simulink model "Lazurit_zarud_"  (R2018b)
settings: Solver=VariableStepAuto  StartTime=0.0  StopTime=1  RelTol=1e-3
undefined symbols (not defined in the file): Cout_c, Cout_filter_c, Cout_filter_r, Cout_r, Czpt_c, Czpt_r, DiscIntNeverNeededParam, f, L_l, L_r, Lzpt_l, Lzpt_r, Rout, Ul, Uout
libraries: powerlib x36, dspstat3 x15, powerlib_meascontrol x8, simulink x4, simulink_extras x4, peRmsMeasurement x4
settings Model: Creator=VID Company  LastModifiedBy=VID Company

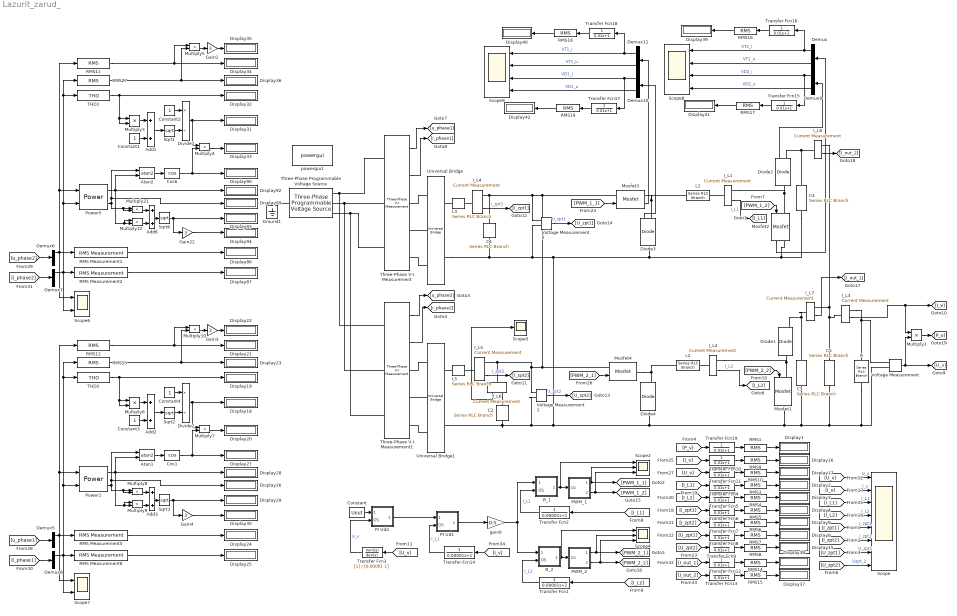
== system Lazurit_zarud_ ==
  Add{1..3,6} (4 alike) : Sum
  Atan1 : Trigonometry  Operator=atan2
  Atan2 : Trigonometry  Operator=atan2
  C1 : powerlib/Elements/Series RLC Branch  LConnTagsString=__new0  RConnTagsString=__new0  BranchType=RC  Resistance=Czpt_r  Inductance=1e-3  SetiL0=off  InitialCurrent=0  Capacitance=Czpt_c  Setx0=on  InitialVoltage=Uzpt  Measurements=Branch voltage
      settings: SourceProductName=Simscape Electrical
  C2 : powerlib/Elements/Series RLC Branch  LConnTagsString=__new0  RConnTagsString=__new0  BranchType=RC  Resistance=Czpt_r  Inductance=1e-3  SetiL0=off  InitialCurrent=0  Capacitance=Czpt_c  Setx0=on  InitialVoltage=Uzpt  Measurements=Branch voltage
      settings: SourceProductName=Simscape Electrical
  C3 : powerlib/Elements/Series RLC Branch  LConnTagsString=__new0  RConnTagsString=__new0  BranchType=RC  Resistance=Cout_r  Inductance=1e-3  SetiL0=off  InitialCurrent=0  Capacitance=Cout_c  Setx0=on  InitialVoltage=0  Measurements=Branch voltage
      settings: SourceProductName=Simscape Electrical
  C4 : powerlib/Elements/Series RLC Branch  LConnTagsString=__new0  RConnTagsString=__new0  BranchType=RC  Resistance=Cout_r  Inductance=1e-3  SetiL0=off  InitialCurrent=0  Capacitance=Cout_c  Setx0=on  InitialVoltage=0  Measurements=Branch voltage
      settings: SourceProductName=Simscape Electrical
  C5 : powerlib/Elements/Series RLC Branch  LConnTagsString=__new0  RConnTagsString=__new0  BranchType=RC  Resistance=Cout_filter_r  Inductance=1e-3  SetiL0=off  InitialCurrent=0  Capacitance=Cout_filter_c  Setx0=on  InitialVoltage=0  Measurements=Branch voltage
      settings: SourceProductName=Simscape Electrical
  Constant : Constant  Value=Uout
  Constant{1..4} (4 alike) : Constant
  Cos1 : Trigonometry  Operator=cos
  Cos6 : Trigonometry  Operator=cos
  Demux{,9..11} (4 alike) : Demux  Outputs=2
  Demux{5..8} (4 alike) : Demux  Outputs=3
  Diode{1..4} (4 alike) : powerlib/Power Electronics/Diode  Ron=0.001  Lon=0  Vf=0.8  IC=0  UseSnubber=off  Rs=500  Cs=250e-9  Measurements=on
      settings: SourceProductName=Simscape Electrical
  Display{1..4,8..9,15..42,86..87,89..90,92..94} (41 alike) : Display
  Divide1 : Product  Inputs=*/
  Divide2 : Product  Inputs=*/
  Gain{1,3..4,22} (4 alike) : Gain  Gain=3
  Ground1 : powerlib/Elements/Ground  LConnTagsString=a
  I_L{1..8} (8 alike) : powerlib/Measurements/Current Measurement  PhasorSimulation=off  OutputType=Complex  PSBequivalent=0
      settings: SourceProductName=Simscape Electrical
  L1 : powerlib/Elements/Series RLC Branch  LConnTagsString=__new0  RConnTagsString=__new0  BranchType=RL  Resistance=L_r  Inductance=L_l  SetiL0=off  InitialCurrent=0  Capacitance=1e-6  Setx0=off  InitialVoltage=0  Measurements=None
      settings: SourceProductName=Simscape Electrical
  L2 : powerlib/Elements/Series RLC Branch  LConnTagsString=__new0  RConnTagsString=__new0  BranchType=RL  Resistance=L_r  Inductance=L_l  SetiL0=off  InitialCurrent=0  Capacitance=1e-6  Setx0=off  InitialVoltage=0  Measurements=None
      settings: SourceProductName=Simscape Electrical
  L3 : powerlib/Elements/Series RLC Branch  LConnTagsString=__new0  RConnTagsString=__new0  BranchType=RL  Resistance=Lzpt_r  Inductance=Lzpt_l  SetiL0=off  InitialCurrent=0  Capacitance=1e-6  Setx0=off  InitialVoltage=0  Measurements=None
      settings: SourceProductName=Simscape Electrical
  L5 : powerlib/Elements/Series RLC Branch  LConnTagsString=__new0  RConnTagsString=__new0  BranchType=RL  Resistance=Lzpt_r  Inductance=Lzpt_l  SetiL0=off  InitialCurrent=0  Capacitance=1e-6  Setx0=off  InitialVoltage=0  Measurements=None
      settings: SourceProductName=Simscape Electrical
  Mosfet1 : powerlib/Power Electronics/Mosfet  Ron=1e-6  Lon=0  Rd=1e-6  Vfd=0  IC=0  Rs=1e5  Cs=inf  Measurements=off
      settings: SourceProductName=Simscape Electrical
  Mosfet2 : powerlib/Power Electronics/Mosfet  Ron=1e-6  Lon=0  Rd=1e-6  Vfd=0  IC=0  Rs=1e5  Cs=inf  Measurements=on
      settings: SourceProductName=Simscape Electrical
  Mosfet3 : powerlib/Power Electronics/Mosfet  Ron=1e-6  Lon=0  Rd=1e-6  Vfd=0  IC=0  Rs=1e5  Cs=inf  Measurements=on
      settings: SourceProductName=Simscape Electrical
  Mosfet4 : powerlib/Power Electronics/Mosfet  Ron=1e-6  Lon=0  Rd=1e-6  Vfd=0  IC=0  Rs=1e5  Cs=inf  Measurements=off
      settings: SourceProductName=Simscape Electrical
  Multiply{1,3..10,21..22} (11 alike) : Product
  PI Ud1 : Subsystem
  PI Ud2 : Subsystem
  PWM_1 : Subsystem
  PWM_2 : Subsystem
  Power1 : powerlib_meascontrol/Measurements/Power  Freq=50  Vinit=[1, 0]  Iinit=[1, 0]  Ts=0
      settings: SourceProductName=Simscape Power Systems
  Power5 : powerlib_meascontrol/Measurements/Power  Freq=50  Vinit=[1, 0]  Iinit=[1, 0]  Ts=0
      settings: SourceProductName=Simscape Power Systems
  R : powerlib/Elements/Series RLC Branch  LConnTagsString=__new0  RConnTagsString=__new0  BranchType=R  Resistance=Rout  Inductance=1e-3  SetiL0=off  InitialCurrent=0  Capacitance=6000e-6  Setx0=off  InitialVoltage=0  Measurements=None
  RMS Measurement{1..2,5,8} (4 alike) : peRmsMeasurement/RMS Measurement  LabelModeActiveChoice=Harmonic  F=50  SpecifyHarmonics=on  K=[1]  Ts=0
  RMS{1,3..10,14..19} (15 alike) : dspstat3/RMS  run=off  directionMode=Each column  dimension=1  InputProcessing=Columns as channels (frame based)  reset_popup=None
  RMS{11..13,27} (4 alike) : powerlib_meascontrol/Measurements/RMS  TrueRMS=on  Freq=50  RMSInit=0  Ts=0
  R_1 : Subsystem
  R_2 : Subsystem
  Scope : Scope  NumInputPorts=8
  Scope2 : Scope  NumInputPorts=3
  Scope4 : Scope  NumInputPorts=3
  Scope5 : Scope
  Scope6 : Scope  NumInputPorts=2
  Scope7 : Scope  NumInputPorts=2
  Scope8 : Scope  NumInputPorts=4
  Scope9 : Scope  NumInputPorts=4
  Sqrt{1..3,6} (4 alike) : Sqrt  SaturateOnIntegerOverflow=on
  THD1 : powerlib_meascontrol/Measurements/THD  Freq=50  Ts=0
  THD2 : powerlib_meascontrol/Measurements/THD  Freq=50  Ts=0
  Three-Phase Programmable Voltage Source : powerlib/Electrical Sources/Three-Phase Programmable Voltage Source  PositiveSequence=[Ul 0 50]  VariationEntity=None  VariationType=Table of time-amplitude pairs  VariationTypeAlt=Step  VariationStep=0.5  VariationRate=10  VariationMagnitude=0.3  VariationFrequency=2  VariationTiming=[1 2]  VariationPhaseA=off  Amplitudes=[1 0.8 1.2 1.0]  TimeValues=[0 0.1 0.15 0.2]  HarmonicGeneration=off  HarmonicA=[3 0.2 -25 0]  HarmonicB=[2 0.15 35 2]  Timing="[0.05  3]"  BusType=swing  Pref=0  Qref=0  Qmin=-inf  Qmax=inf
  Three-Phase V-I Measurement : powerlib/Measurements/Three-Phase V-I Measurement  VoltageMeasurement=phase-to-ground  SetLabelV=off  LabelV=Vabc  Vpu=off  VpuLL=off  CurrentMeasurement=yes  SetLabelI=off  LabelI=Iabc  Ipu=off  Pbase=100e6  Vbase=500e3  OutputType=Complex  PhasorSimulation=off  PSBequivalent=0
  Three-Phase V-I Measurement1 : powerlib/Measurements/Three-Phase V-I Measurement  VoltageMeasurement=phase-to-ground  SetLabelV=off  LabelV=Vabc  Vpu=off  VpuLL=off  CurrentMeasurement=yes  SetLabelI=off  LabelI=Iabc  Ipu=off  Pbase=100e6  Vbase=500e3  OutputType=Complex  PhasorSimulation=off  PSBequivalent=0
  Transfer Fcn{1..3,14} (4 alike) : TransferFcn  Denominator=[0.00001 1]
  Transfer Fcn{4..13,15..19} (15 alike) : TransferFcn  Denominator=[0.01 1]
  Universal Bridge : powerlib/Power Electronics/Universal Bridge  Arms=3  SnubberResistance=1e5  SnubberCapacitance=inf  Device=Diodes  Ron=Vd_r  Lon=0  ForwardVoltages="[  0  0  ]"  ForwardVoltage=Vd_v  GTOparameters=[ 10e-6 , 20e-6 ]  IGBTparameters=[ 1e-6 , 2e-6 ]  Measurements=None  Measurements_2=None  converterType=Rectifier
  Universal Bridge1 : powerlib/Power Electronics/Universal Bridge  Arms=3  SnubberResistance=1e5  SnubberCapacitance=inf  Device=Diodes  Ron=Vd_r  Lon=0  ForwardVoltages="[  0  0  ]"  ForwardVoltage=Vd_v  GTOparameters=[ 10e-6 , 20e-6 ]  IGBTparameters=[ 1e-6 , 2e-6 ]  Measurements=None  Measurements_2=None  converterType=Rectifier
  Voltage Measurement : powerlib/Measurements/Voltage Measurement  PhasorSimulation=off  OutputType=Complex  PSBequivalent=0
  Voltage Measurement1 : powerlib/Measurements/Voltage Measurement  PhasorSimulation=off  OutputType=Complex  PSBequivalent=0
  Voltage Measurement2 : powerlib/Measurements/Voltage Measurement  PhasorSimulation=off  OutputType=Complex  PSBequivalent=0
  gain6 : Gain  Gain=0.5  SaturateOnIntegerOverflow=on  OutDataTypeStr=Inherit: Same as input  ParamDataTypeStr=Inherit: Same as input
  powergui1 : powerlib/powergui  Priority=1  SimulationMode=Discrete  SampleTime=1e-6  frequency=60  Iterations=50  frequencyindice=50  Pbase=100e6  ErrMax=1e-4  UnitsV=kV  UnitsW=MW  buscounter=0  FunctionMessages=off  echomessages=off  EnableUseOfTLC=off  CurrentSourceSwitches=off  DisableSnubberDevices=off  DisableRonSwitches=off  DisableVfSwitches=off  DisplayEquations=off  SolverType=Tustin/Backward Euler (TBE)  Interpol=off  ExternalGateDelay=off  methode=off  Ts=100  x0status=blocks  SPID=on  SwTol=0  HookPort=off  RestoreLinks=warning  ResistiveCurrentMeasurement=off  Frange=[0:2:500]  Ylog=off  Xlog=on  ShowGrid=off  save=off  variable=ZData  structure=logsout  ZoomFFT=off  StartTime=0.1  cycles=30  DisplayStyle=2  fundamental=50  FreqAxis=off  MaxFrequency=1000  frequencyindicesteady=1  RmsSteady=1  display=off
  wires:
  Three-Phase V-I Measurement/1 -> [u_phase1]
  Three-Phase V-I Measurement1/1 -> [u_phase2]
  Three-Phase V-I Measurement/2 -> [i_phase1]
  Three-Phase V-I Measurement1/2 -> [i_phase2]
  R_1/1(Out) -> Scope2/1, PWM_1/1(Uz)
  Transfer Fcn2/1 -> R_1/2(OS)  "I_L1"
  Transfer Fcn1/1 -> R_2/2(OS)  "I_L2"
  gain6/1 -> R_1/1(Zad), R_2/1(Zad)
  R_2/1(Out) -> Scope4/1, PWM_2/1(Uz)
  Constant/1 -> PI Ud2/1(Zad)
  Transfer Fcn3/1 -> PI Ud2/2(OS)  "U_v"
  I_L1/1 -> [I_L1]  "I_L1"
  PWM_1/1(CH1) -> Scope2/2, [PWM_1_1]
  [PWM_1_2] -> Mosfet2/1
  [I_L1] -> Transfer Fcn2/1
  PWM_2/1(CH1) -> Scope4/2, [PWM_2_1]
  I_L2/1 -> [I_L2]  "I_L2"
  [I_L2] -> Transfer Fcn1/1
  [PWM_2_2] -> Mosfet1/1
  Voltage Measurement/1 -> [U_v], Multiply1/2
  [U_v] -> Transfer Fcn3/1
  [U_v] -> Scope/1  "U_v"
  [I_L1] -> Scope/3  "I_L1"
  [I_L2] -> Scope/4  "I_L2"
  I_L3/1 -> [I_v], Multiply1/1
  [I_v] -> Scope/2  "I_v"
  I_L5/1 -> [I_zpt2]  "I_zpt2"
  I_L4/1 -> [I_zpt1]  "I_zpt1"
  [I_zpt1] -> Scope/5  "I_zpt1"
  [I_zpt2] -> Scope/6  "I_zpt2"
  Voltage Measurement1/1 -> [U_zpt2]  "U_zpt2"
  Voltage Measurement2/1 -> [U_zpt1]  "U_zpt1"
  [U_zpt1] -> Scope/7  "U_zpt1"
  [U_zpt2] -> Scope/8  "Uzpt_2"
  Multiply1/1 -> [P_v]
  [I_L1] -> Transfer Fcn4/1
  [I_L2] -> Transfer Fcn5/1
  [I_zpt1] -> Transfer Fcn6/1
  [I_zpt2] -> Transfer Fcn7/1
  [U_zpt1] -> Transfer Fcn8/1
  [U_zpt2] -> Transfer Fcn9/1
  RMS3/1 -> Display2/1
  RMS4/1 -> Display3/1
  RMS5/1 -> Display4/1
  RMS6/1 -> Display9/1
  RMS7/1 -> Display8/1
  RMS8/1 -> Display15/1
  Transfer Fcn4/1 -> RMS3/1
  Transfer Fcn5/1 -> RMS4/1
  Transfer Fcn6/1 -> RMS5/1
  Transfer Fcn7/1 -> RMS6/1
  Transfer Fcn8/1 -> RMS7/1
  Transfer Fcn9/1 -> RMS8/1
  PWM_1/2(CH2) -> Scope2/3, [PWM_1_2]
  [PWM_1_1] -> Mosfet3/1
  PWM_2/2(CH2) -> [PWM_2_2], Scope4/3
  [PWM_2_1] -> Mosfet4/1
  Transfer Fcn10/1 -> RMS9/1
  RMS9/1 -> Display16/1
  [I_v] -> Transfer Fcn10/1
  Transfer Fcn11/1 -> RMS10/1
  RMS10/1 -> Display17/1
  [U_v] -> Transfer Fcn11/1
  I_L6/1 -> Scope5/1
  Multiply3/1 -> Add1/1
  Multiply5/1 -> Gain1/1
  Add1/1 -> Sqrt1/1
  Multiply4/1 -> Display33/1
  Constant1/1 -> Add1/2
  Constant2/1 -> Divide1/1
  Power5/1 -> Atan2/2, Multiply22/1, Multiply22/2, Display92/1
  Cos6/1 -> Multiply4/2, Display90/1
  RMS Measurement1/1 -> Display86/1
  Demux7/1 -> Scope6/2, RMS Measurement2/1, THD1/1, RMS27/1, Power5/2
  [i_phase2] -> Demux7/1
  Power5/2 -> Atan2/1, Display89/1, Multiply21/2, Multiply21/1
  [i_phase1] -> Demux8/1
  RMS11/1 -> Multiply5/1, Display34/1
  Sqrt2/1 -> Divide2/2
  Gain1/1 -> Display35/1
  Multiply21/1 -> Add6/1
  Divide1/1 -> Multiply4/1, Display31/1
  Demux6/1 -> Scope6/1, RMS Measurement1/1, RMS11/1, Power5/1
  Cos1/1 -> Multiply7/2, Display27/1
  Gain3/1 -> Display22/1
  Multiply8/1 -> Add3/1
  Multiply9/1 -> Add3/2
  Sqrt6/1 -> Display93/1, Gain22/1
  Sqrt1/1 -> Divide1/2
  Divide2/1 -> Multiply7/1, Display18/1
  [u_phase2] -> Demux6/1
  Atan2/1 -> Cos6/1
  Add6/1 -> Sqrt6/1
  RMS Measurement8/1 -> Display25/1
  Atan1/1 -> Cos1/1
  RMS Measurement5/1 -> Display24/1
  Demux8/1 -> Scope7/2, RMS Measurement8/1, THD2/1, RMS13/1, Power1/2
  [u_phase1] -> Demux5/1
  Constant4/1 -> Divide2/1
  RMS13/1 -> Multiply10/2, Display23/1
  RMS Measurement2/1 -> Display87/1
  RMS12/1 -> Multiply10/1, Display21/1
  Multiply6/1 -> Add2/1
  Gain4/1 -> Display30/1
  RMS27/1 -> Multiply5/2, Display36/1
  THD1/1 -> Multiply3/2, Multiply3/1, Display32/1
  Sqrt3/1 -> Display29/1, Gain4/1
  Power1/2 -> Atan1/1, Display26/1, Multiply8/2, Multiply8/1
  Add2/1 -> Sqrt2/1
  Gain22/1 -> Display94/1
  THD2/1 -> Multiply6/2, Multiply6/1, Display19/1
  Demux5/1 -> Scope7/1, RMS Measurement5/1, RMS12/1, Power1/1
  Power1/1 -> Atan1/2, Multiply9/1, Multiply9/2, Display28/1
  Multiply22/1 -> Add6/2
  Constant3/1 -> Add2/2
  Add3/1 -> Sqrt3/1
  Multiply10/1 -> Gain3/1
  Multiply7/1 -> Display20/1
  I_L7/1 -> [I_out_1]
  I_L8/1 -> [I_out_2]
  [I_out_2] -> Transfer Fcn13/1
  [I_out_1] -> Transfer Fcn12/1
  Transfer Fcn12/1 -> RMS14/1
  RMS14/1 -> Display38/1
  Transfer Fcn13/1 -> RMS15/1
  RMS15/1 -> Display37/1
  PI Ud1/1(Out) -> gain6/1
  PI Ud2/1(Out) -> PI Ud1/1(Zad)
  [I_v] -> Transfer Fcn14/1
  Transfer Fcn14/1 -> PI Ud1/2(OS)  "I_L1"
  Mosfet2/1 -> Demux/1
  Demux/1 -> Transfer Fcn16/1, Scope8/1  "VT2_i"
  Demux/2 -> Scope8/2  "VT2_u"
  Demux9/1 -> Scope8/3, Transfer Fcn15/1  "VD2_i"
  Demux9/2 -> Scope8/4  "VD2_u"
  Diode2/1 -> Demux9/1
  Transfer Fcn16/1 -> RMS16/1
  RMS16/1 -> Display39/1
  Transfer Fcn15/1 -> RMS17/1
  RMS17/1 -> Display41/1
  Mosfet3/1 -> Demux11/1
  Diode3/1 -> Demux10/1
  Demux10/2 -> Scope9/4  "VD1_u"
  Demux11/1 -> Transfer Fcn18/1, Scope9/1  "VT1_i"
  Demux10/1 -> Scope9/3, Transfer Fcn17/1  "VD1_i"
  Transfer Fcn18/1 -> RMS18/1
  Demux11/2 -> Scope9/2  "VT1_u"
  Transfer Fcn17/1 -> RMS19/1
  RMS18/1 -> Display40/1
  RMS19/1 -> Display42/1
  Transfer Fcn19/1 -> RMS1/1
  RMS1/1 -> Display1/1
  [P_v] -> Transfer Fcn19/1
  connections:
  Three-Phase Programmable Voltage Source/RConn3 -- Three-Phase V-I Measurement1/LConn3 -- Three-Phase V-I Measurement/LConn3
  Three-Phase Programmable Voltage Source/RConn1 -- Three-Phase V-I Measurement1/LConn1 -- Three-Phase V-I Measurement/LConn1
  Three-Phase Programmable Voltage Source/RConn2 -- Three-Phase V-I Measurement1/LConn2 -- Three-Phase V-I Measurement/LConn2
  Three-Phase Programmable Voltage Source/LConn1 -- Ground1/LConn1
  Universal Bridge/LConn1 -- Three-Phase V-I Measurement/RConn1
  Universal Bridge/LConn2 -- Three-Phase V-I Measurement/RConn2
  Universal Bridge/LConn3 -- Three-Phase V-I Measurement/RConn3
  I_L3/RConn1 -- R/LConn1 -- Voltage Measurement/LConn1
  Diode2/LConn1 -- Mosfet2/LConn1 -- I_L1/RConn1
  Mosfet1/LConn1 -- I_L2/RConn1 -- Diode1/LConn1
  I_L1/LConn1 -- L1/RConn1
  I_L2/LConn1 -- L2/RConn1
  C3/LConn1 -- I_L7/LConn1 -- Diode1/RConn1
  L3/LConn1 -- Universal Bridge/RConn1
  L5/LConn1 -- Universal Bridge1/RConn1
  Mosfet3/RConn1 -- Diode3/RConn1 -- L1/LConn1
  Universal Bridge1/LConn1 -- Three-Phase V-I Measurement1/RConn1
  Universal Bridge1/LConn2 -- Three-Phase V-I Measurement1/RConn2
  Universal Bridge1/LConn3 -- Three-Phase V-I Measurement1/RConn3
  Mosfet4/LConn1 -- I_L5/RConn1 -- I_L6/LConn1 -- Voltage Measurement1/LConn1 -- Mosfet3/LConn1 -- C1/LConn1 -- I_L4/RConn1 -- Voltage Measurement2/LConn1
  I_L5/LConn1 -- L5/RConn1
  I_L4/LConn1 -- L3/RConn1
  Mosfet4/RConn1 -- L2/LConn1 -- Diode4/RConn1
  Voltage Measurement1/LConn2 -- Universal Bridge1/RConn2 -- C2/RConn1 -- Diode3/LConn1 -- C4/RConn1 -- Mosfet2/RConn1 -- Voltage Measurement2/LConn2 -- Universal Bridge/RConn2 -- C1/RConn1 -- Mosfet1/RConn1 -- C5/RConn1 -- Voltage Measurement/LConn2 -- R/RConn1 -- C3/RConn1 -- Diode4/LConn1
  I_L6/RConn1 -- C2/LConn1
  C5/LConn1 -- I_L8/RConn1 -- I_L7/RConn1 -- I_L3/LConn1
  Diode2/RConn1 -- I_L8/LConn1 -- C4/LConn1

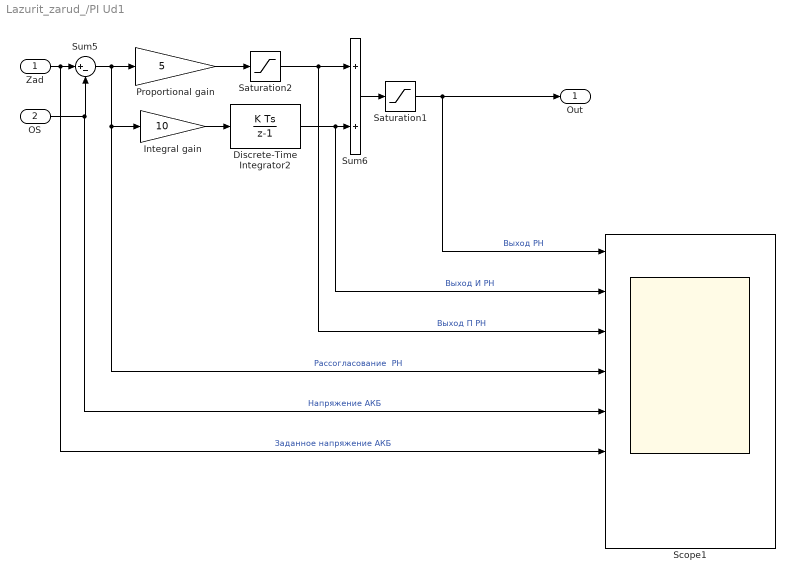
== system Lazurit_zarud_/PI Ud1 ==
  Zad : Inport
  OS : Inport  Port=2
  Discrete-Time Integrator2 : DiscreteIntegrator  SampleTime=-1  LimitOutput=on  UpperSaturationLimit=260  LowerSaturationLimit=0  ICPrevOutput=DiscIntNeverNeededParam  ICPrevScaledInput=DiscIntNeverNeededParam
  Integral gain : Gain  Gain=10  SaturateOnIntegerOverflow=on  OutDataTypeStr=Inherit: Same as input  ParamDataTypeStr=Inherit: Same as input
  Proportional gain : Gain  Gain=5  SaturateOnIntegerOverflow=on  OutDataTypeStr=Inherit: Same as input  ParamDataTypeStr=Inherit: Same as input
  Saturation1 : Saturate  UpperLimit=260  LowerLimit=0
  Saturation2 : Saturate  UpperLimit=260  LowerLimit=-260
  Scope1 : Scope  NumInputPorts=8
  Sum5 : Sum  Inputs=|+-  SaturateOnIntegerOverflow=on  InputSameDT=on  OutDataTypeStr=Inherit: Same as first input
  Sum6 : Sum  SaturateOnIntegerOverflow=on  InputSameDT=on  OutDataTypeStr=Inherit: Same as first input
  Out : Outport
  wires:
  Integral gain/1 -> Discrete-Time Integrator2/1
  Discrete-Time Integrator2/1 -> Scope1/2, Sum6/2  "Выход И РН"
  OS/1 -> Scope1/5, Sum5/2  "Напряжение АКБ"
  Zad/1 -> Scope1/6, Sum5/1  "Заданное напряжение АКБ"
  Sum5/1 -> Scope1/4, Integral gain/1, Proportional gain/1  "Рассогласование  РН"
  Sum6/1 -> Saturation1/1
  Saturation1/1 -> Out/1, Scope1/1  "Выход РН"
  Proportional gain/1 -> Saturation2/1
  Saturation2/1 -> Scope1/3, Sum6/1  "Выход П РН"

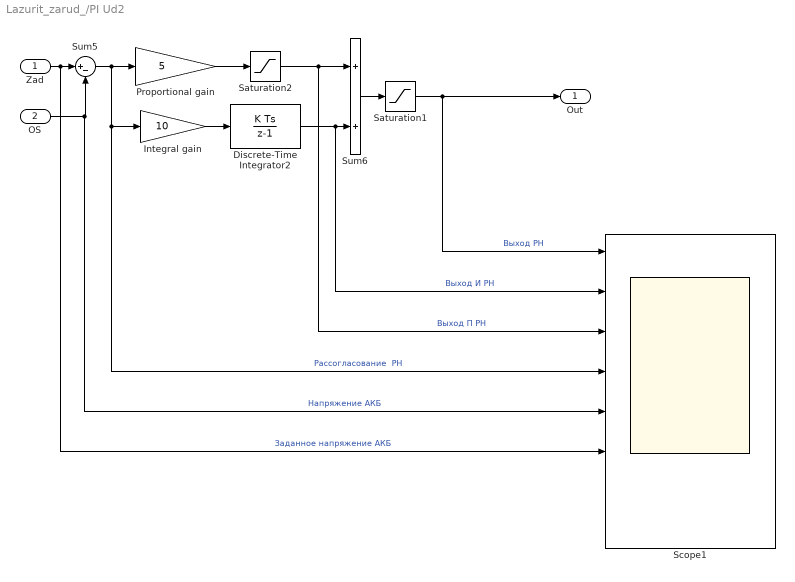
== system Lazurit_zarud_/PI Ud2 ==
  Zad : Inport
  OS : Inport  Port=2
  Discrete-Time Integrator2 : DiscreteIntegrator  SampleTime=-1  LimitOutput=on  UpperSaturationLimit=250  LowerSaturationLimit=0  ICPrevOutput=DiscIntNeverNeededParam  ICPrevScaledInput=DiscIntNeverNeededParam
  Integral gain : Gain  Gain=10  SaturateOnIntegerOverflow=on  OutDataTypeStr=Inherit: Same as input  ParamDataTypeStr=Inherit: Same as input
  Proportional gain : Gain  Gain=5  SaturateOnIntegerOverflow=on  OutDataTypeStr=Inherit: Same as input  ParamDataTypeStr=Inherit: Same as input
  Saturation1 : Saturate  UpperLimit=250  LowerLimit=0
  Saturation2 : Saturate  UpperLimit=250  LowerLimit=-250
  Scope1 : Scope  NumInputPorts=8
  Sum5 : Sum  Inputs=|+-  SaturateOnIntegerOverflow=on  InputSameDT=on  OutDataTypeStr=Inherit: Same as first input
  Sum6 : Sum  SaturateOnIntegerOverflow=on  InputSameDT=on  OutDataTypeStr=Inherit: Same as first input
  Out : Outport
  wires:
  Integral gain/1 -> Discrete-Time Integrator2/1
  Discrete-Time Integrator2/1 -> Scope1/2, Sum6/2  "Выход И РН"
  OS/1 -> Scope1/5, Sum5/2  "Напряжение АКБ"
  Zad/1 -> Scope1/6, Sum5/1  "Заданное напряжение АКБ"
  Sum5/1 -> Scope1/4, Integral gain/1, Proportional gain/1  "Рассогласование  РН"
  Sum6/1 -> Saturation1/1
  Saturation1/1 -> Out/1, Scope1/1  "Выход РН"
  Proportional gain/1 -> Saturation2/1
  Saturation2/1 -> Scope1/3, Sum6/1  "Выход П РН"

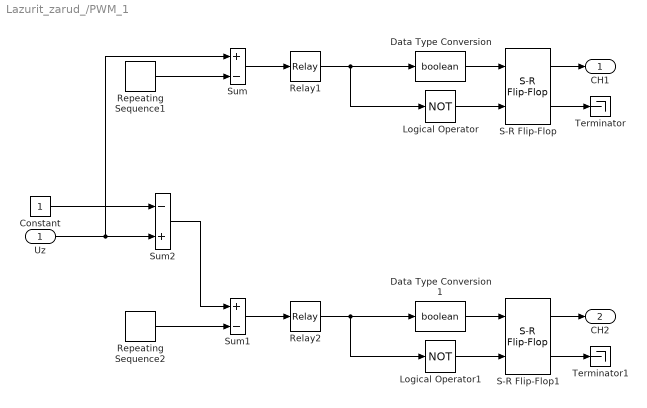
== system Lazurit_zarud_/PWM_1 ==
  Uz : Inport
  Constant : Constant
  Data Type Conversion : DataTypeConversion  OutDataTypeStr=boolean
  Data Type Conversion1 : DataTypeConversion  OutDataTypeStr=boolean
  Logical Operator : Logic  Operator=NOT  AllPortsSameDT=off  OutDataTypeStr=boolean
  Logical Operator1 : Logic  Operator=NOT  AllPortsSameDT=off  OutDataTypeStr=boolean
  Relay1 : Relay  OnSwitchValue=0.01  OffSwitchValue=-0.01
  Relay2 : Relay  OnSwitchValue=0.01  OffSwitchValue=-0.01
  Repeating Sequence1 : simulink/Sources/Repeating Sequence  rep_seq_t="[0  (1/(2*f)) (1/f)]"  rep_seq_y=[0 1 0]
  Repeating Sequence2 : simulink/Sources/Repeating Sequence  rep_seq_t="[0  (1/(2*f)) (1/f)]"  rep_seq_y=[0 1 0]
  S-R Flip-Flop : simulink_extras/Flip Flops/S-R Flip-Flop  initial_condition=0
  S-R Flip-Flop1 : simulink_extras/Flip Flops/S-R Flip-Flop  initial_condition=0
  Sum : Sum  Inputs=+-
  Sum1 : Sum  Inputs=+-
  Sum2 : Sum  Inputs=-+
  Terminator : Terminator
  Terminator1 : Terminator
  CH1 : Outport
  CH2 : Outport  Port=2
  wires:
  S-R Flip-Flop/1 -> CH1/1
  Data Type Conversion/1 -> S-R Flip-Flop/1
  Logical Operator/1 -> S-R Flip-Flop/2
  Relay1/1 -> Logical Operator/1, Data Type Conversion/1
  Repeating Sequence1/1 -> Sum/2
  Sum/1 -> Relay1/1
  S-R Flip-Flop/2 -> Terminator/1
  Data Type Conversion1/1 -> S-R Flip-Flop1/1
  Logical Operator1/1 -> S-R Flip-Flop1/2
  S-R Flip-Flop1/2 -> Terminator1/1
  Relay2/1 -> Logical Operator1/1, Data Type Conversion1/1
  S-R Flip-Flop1/1 -> CH2/1
  Sum1/1 -> Relay2/1
  Uz/1 -> Sum/1, Sum2/2
  Constant/1 -> Sum2/1
  Sum2/1 -> Sum1/1
  Repeating Sequence2/1 -> Sum1/2

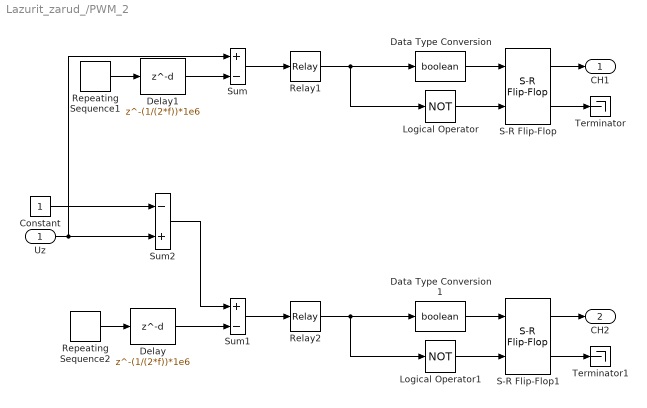
== system Lazurit_zarud_/PWM_2 ==
  Uz : Inport
  Constant : Constant
  Data Type Conversion : DataTypeConversion  OutDataTypeStr=boolean
  Data Type Conversion1 : DataTypeConversion  OutDataTypeStr=boolean
  Delay : Delay  DelayLength=(1/(2*f))*1e6
  Delay1 : Delay  DelayLength=(1/(2*f))*1e6
  Logical Operator : Logic  Operator=NOT  AllPortsSameDT=off  OutDataTypeStr=boolean
  Logical Operator1 : Logic  Operator=NOT  AllPortsSameDT=off  OutDataTypeStr=boolean
  Relay1 : Relay  OnSwitchValue=0.01  OffSwitchValue=-0.01
  Relay2 : Relay  OnSwitchValue=0.01  OffSwitchValue=-0.01
  Repeating Sequence1 : simulink/Sources/Repeating Sequence  rep_seq_t="[0  (1/(2*f)) (1/f)]"  rep_seq_y=[0 1 0]
  Repeating Sequence2 : simulink/Sources/Repeating Sequence  rep_seq_t="[0  (1/(2*f)) (1/f)]"  rep_seq_y=[0 1 0]
  S-R Flip-Flop : simulink_extras/Flip Flops/S-R Flip-Flop  initial_condition=0
  S-R Flip-Flop1 : simulink_extras/Flip Flops/S-R Flip-Flop  initial_condition=0
  Sum : Sum  Inputs=+-
  Sum1 : Sum  Inputs=+-
  Sum2 : Sum  Inputs=-+
  Terminator : Terminator
  Terminator1 : Terminator
  CH1 : Outport
  CH2 : Outport  Port=2
  wires:
  S-R Flip-Flop/1 -> CH1/1
  Data Type Conversion/1 -> S-R Flip-Flop/1
  Logical Operator/1 -> S-R Flip-Flop/2
  Relay1/1 -> Logical Operator/1, Data Type Conversion/1
  Sum/1 -> Relay1/1
  S-R Flip-Flop/2 -> Terminator/1
  Data Type Conversion1/1 -> S-R Flip-Flop1/1
  Logical Operator1/1 -> S-R Flip-Flop1/2
  S-R Flip-Flop1/2 -> Terminator1/1
  Relay2/1 -> Logical Operator1/1, Data Type Conversion1/1
  S-R Flip-Flop1/1 -> CH2/1
  Sum1/1 -> Relay2/1
  Repeating Sequence2/1 -> Delay/1
  Uz/1 -> Sum2/2, Sum/1
  Constant/1 -> Sum2/1
  Sum2/1 -> Sum1/1
  Delay/1 -> Sum1/2
  Repeating Sequence1/1 -> Delay1/1
  Delay1/1 -> Sum/2

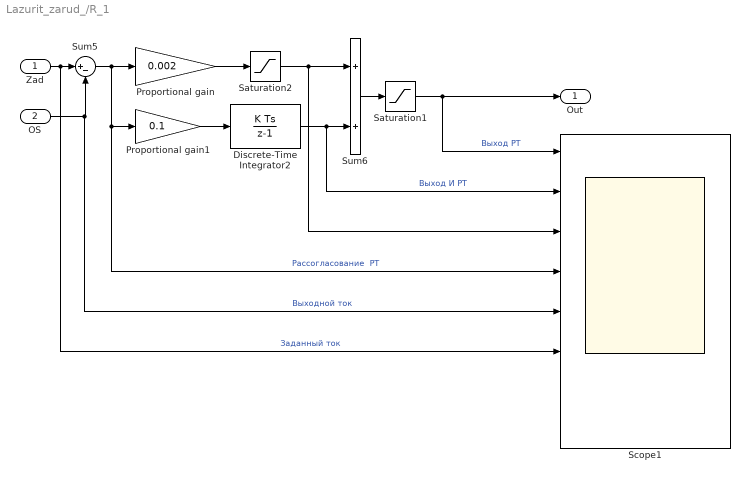
== system Lazurit_zarud_/R_1 ==
  Zad : Inport
  OS : Inport  Port=2
  Discrete-Time Integrator2 : DiscreteIntegrator  SampleTime=-1  LimitOutput=on  UpperSaturationLimit=1.35  LowerSaturationLimit=0  ICPrevOutput=DiscIntNeverNeededParam  ICPrevScaledInput=DiscIntNeverNeededParam
  Proportional gain : Gain  Gain=0.002  SaturateOnIntegerOverflow=on  OutDataTypeStr=Inherit: Same as input  ParamDataTypeStr=Inherit: Same as input
  Proportional gain1 : Gain  Gain=0.1  SaturateOnIntegerOverflow=on  OutDataTypeStr=Inherit: Same as input  ParamDataTypeStr=Inherit: Same as input
  Saturation1 : Saturate  UpperLimit=1.35  LowerLimit=0
  Saturation2 : Saturate  UpperLimit=0.8  LowerLimit=-0.8
  Scope1 : Scope  NumInputPorts=8
  Sum5 : Sum  Inputs=|+-  SaturateOnIntegerOverflow=on  InputSameDT=on  OutDataTypeStr=Inherit: Same as first input
  Sum6 : Sum  SaturateOnIntegerOverflow=on  InputSameDT=on  OutDataTypeStr=Inherit: Same as first input
  Out : Outport
  wires:
  Proportional gain/1 -> Saturation2/1
  Discrete-Time Integrator2/1 -> Sum6/2, Scope1/2  "Выход И РТ"
  OS/1 -> Scope1/5, Sum5/2  "Выходной ток"
  Zad/1 -> Scope1/6, Sum5/1  "Заданный ток"
  Sum5/1 -> Proportional gain1/1, Scope1/4, Proportional gain/1  "Рассогласование  РТ"
  Sum6/1 -> Saturation1/1
  Saturation1/1 -> Out/1, Scope1/1  "Выход РТ"
  Proportional gain1/1 -> Discrete-Time Integrator2/1
  Saturation2/1 -> Scope1/3, Sum6/1

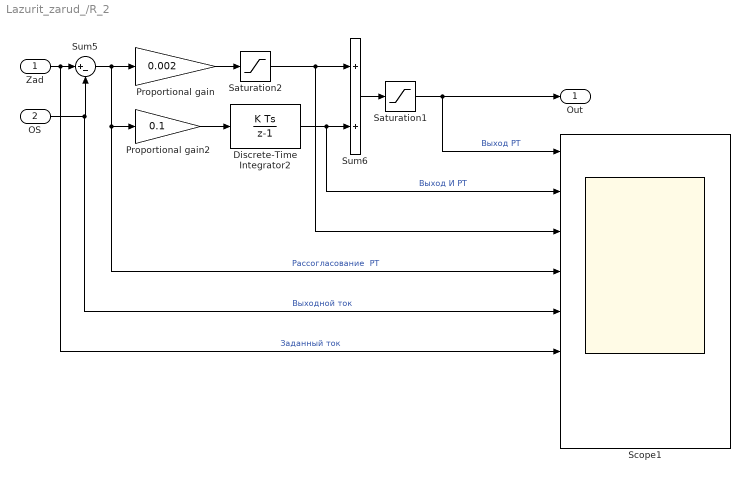
== system Lazurit_zarud_/R_2 ==
  Zad : Inport
  OS : Inport  Port=2
  Discrete-Time Integrator2 : DiscreteIntegrator  SampleTime=-1  LimitOutput=on  UpperSaturationLimit=1.35  LowerSaturationLimit=0  ICPrevOutput=DiscIntNeverNeededParam  ICPrevScaledInput=DiscIntNeverNeededParam
  Proportional gain : Gain  Gain=0.002  SaturateOnIntegerOverflow=on  OutDataTypeStr=Inherit: Same as input  ParamDataTypeStr=Inherit: Same as input
  Proportional gain2 : Gain  Gain=0.1  SaturateOnIntegerOverflow=on  OutDataTypeStr=Inherit: Same as input  ParamDataTypeStr=Inherit: Same as input
  Saturation1 : Saturate  UpperLimit=1.35  LowerLimit=0
  Saturation2 : Saturate  UpperLimit=0.8  LowerLimit=-0.8
  Scope1 : Scope  NumInputPorts=8
  Sum5 : Sum  Inputs=|+-  SaturateOnIntegerOverflow=on  InputSameDT=on  OutDataTypeStr=Inherit: Same as first input
  Sum6 : Sum  SaturateOnIntegerOverflow=on  InputSameDT=on  OutDataTypeStr=Inherit: Same as first input
  Out : Outport
  wires:
  Proportional gain/1 -> Saturation2/1
  Discrete-Time Integrator2/1 -> Sum6/2, Scope1/2  "Выход И РТ"
  OS/1 -> Scope1/5, Sum5/2  "Выходной ток"
  Zad/1 -> Scope1/6, Sum5/1  "Заданный ток"
  Sum5/1 -> Proportional gain2/1, Scope1/4, Proportional gain/1  "Рассогласование  РТ"
  Sum6/1 -> Saturation1/1
  Saturation1/1 -> Out/1, Scope1/1  "Выход РТ"
  Proportional gain2/1 -> Discrete-Time Integrator2/1
  Saturation2/1 -> Scope1/3, Sum6/1
